simulink library "veh"  (Simulink 8.1)
settings: Solver=ode1  StartTime=0.0  StopTime=Inf  FixedStep=0.001  RelTol=1e-3
PostLoadFcn:
  | , if any(exist('dsrtsu_mdlpostloadfcn', 'file') == [2, 3, 6]), try dsrtsu_mdlpostloadfcn('Execute', bdroot); catch fprintf('Error in PostLoadFcn (dsrtsu_mdlpostloadfcn) for model "%s":\n %s\n', bdroot, lasterr); end, end,
undefined symbols (not defined in the file or in its folder): FALSE, KIFO_ACCRelSpeedNoTargets_kph, KIFO_LongAccelNoTargets_mps2, KIFO_RelSpeedNoTargets_kph, KIFO_TargetIdNoTargets_num, KIFO_XPositionNoTargets_m
libraries: hcu_lib x3, aco x1, mcs x1, vec x1, gim x1
settings Model: DSRTSU_INTERNAL_RTI_VER=450  DSRTSU_INTERNAL_RTI_TYPE=rti1401  RTICANMMDATA=struct('GeneralSetupData',struct('modelroot','D:\Projects\ELN150201\Repositories\Taiwan\trunk\AdasDragon\software\sw_development\arch\app\ifo','generalsettings',struct('filesettings',struct('destfolder',struct('Name','RTICANMM_FILES','Check',1),'buildfolder',struct('Name','.','Check',1),'AbsDestfolder',struct('Name','D:\Projects\ELN150201\Repositories\Taiwan\trunk\AdasDragon\software\sw_development\arch\app\ifo\RTICANMM_FILES'),'AbsBuildfolder',struct('Name','D:\Projects\ELN150201\Repositories\Taiwan\trunk\AdasDragon\software\sw_development\arch\app\ifo'))),'options',struct('addpaths',1,'rmpaths',1,'addtrcexclusion',logical(1),'cannavigator',struct('checkmonitoring',0),'show_usrtrc',0,'use_usrtrc',0),'advanced',struct('options',[1 1 1 1 1 1 1 1 1 1 1 1 1 1 1 1 1 1 1 1 1 1 1 1 1 1 1 1 1 1 1 1 1 1 1 1 1 1 1 1 1 1 1 1 1 1 1 1 1 1 1 1 1 1 1 1 1 1 1 1 1 1 1 1 1 1 1 1 1 1 1 1 1 1 1 1 1 1 1 1 1 1 1 1 1 1 1 1 1 1 1 1 1 1 1 1 1 1 1 1]),'MPSetup',{{}},'modelname','veh','block','veh'))  DSRTSU_INTERNAL_RTIFPGA=40  Creator=tescamilla  LastModifiedBy=AT015086

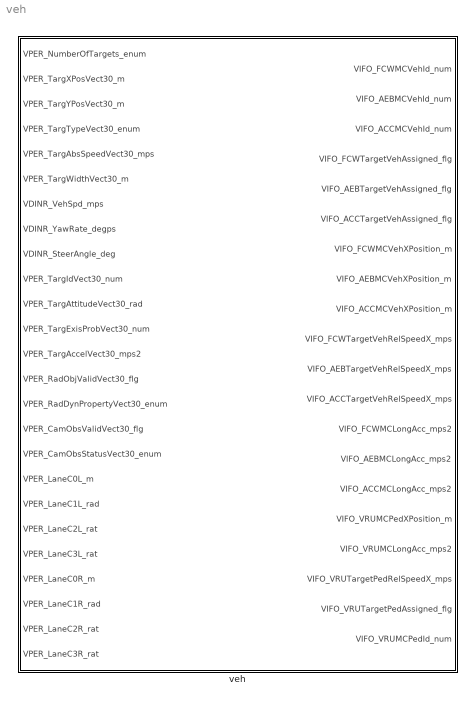
== system veh ==
  veh : Subsystem

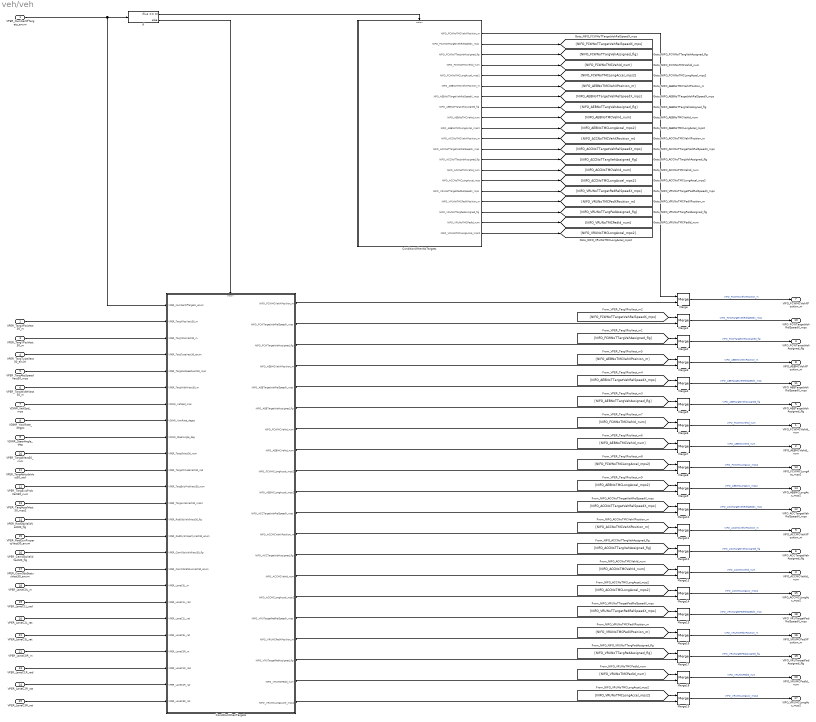
== system veh/veh ==
  VPER_NumberOfTargets_enum : Inport
  VPER_TargXPosVect30_m : Inport  Port=2
  VPER_TargYPosVect30_m : Inport  Port=3
  VPER_TargTypeVect30_enum : Inport  Port=4
  VPER_TargAbsSpeedVect30_mps : Inport  Port=5
  VPER_TargWidthVect30_m : Inport  Port=6
  VDINR_VehSpd_mps : Inport  Port=7
  VDINR_YawRate_degps : Inport  Port=8
  VDINR_SteerAngle_deg : Inport  Port=9
  VPER_TargIdVect30_num : Inport  Port=10
  VPER_TargAttitudeVect30_rad : Inport  Port=11
  VPER_TargExisProbVect30_num : Inport  Port=12
  VPER_TargAccelVect30_mps2 : Inport  Port=13
  VPER_RadObjValidVect30_flg : Inport  Port=14
  VPER_RadDynPropertyVect30_enum : Inport  Port=15
  VPER_CamObsValidVect30_flg : Inport  Port=16
  VPER_CamObsStatusVect30_enum : Inport  Port=17
  VPER_LaneC0L_m : Inport  Port=18
  VPER_LaneC1L_rad : Inport  Port=19
  VPER_LaneC2L_rat : Inport  Port=20
  VPER_LaneC3L_rat : Inport  Port=21
  VPER_LaneC0R_m : Inport  Port=22
  VPER_LaneC1R_rad : Inport  Port=23
  VPER_LaneC2R_rat : Inport  Port=24
  VPER_LaneC3R_rat : Inport  Port=25
  ConditionWhenNoTargets : Subsystem  TreatAsAtomicUnit=on
  ConditionWhenTargets : Subsystem  TreatAsAtomicUnit=on
  If : If  IfExpression=u1 == 0
  Merge : Merge  InitialOutput=KIFO_XPositionNoTargets_m
  Merge1 : Merge  InitialOutput=KIFO_RelSpeedNoTargets_kph
  Merge{6..19} (14 alike) : Merge  InitialOutput=KIFO_TargetIdNoTargets_num
  Merge2 : Merge  InitialOutput=FALSE
  Merge3 : Merge  InitialOutput=KIFO_XPositionNoTargets_m
  Merge4 : Merge  InitialOutput=KIFO_RelSpeedNoTargets_kph
  Merge5 : Merge  InitialOutput=FALSE
  VIFO_FCWMCVehId_num : Outport
  VIFO_AEBMCVehId_num : Outport  Port=2
  VIFO_ACCMCVehId_num : Outport  Port=3
  VIFO_FCWTargetVehAssigned_flg : Outport  Port=4
  VIFO_AEBTargetVehAssigned_flg : Outport  Port=5
  VIFO_ACCTargetVehAssigned_flg : Outport  Port=6
  VIFO_FCWMCVehXPosition_m : Outport  Port=7
  VIFO_AEBMCVehXPosition_m : Outport  Port=8
  VIFO_ACCMCVehXPosition_m : Outport  Port=9
  VIFO_FCWTargetVehRelSpeedX_mps : Outport  Port=10
  VIFO_AEBTargetVehRelSpeedX_mps : Outport  Port=11
  VIFO_ACCTargetVehRelSpeedX_mps : Outport  Port=12
  VIFO_FCWMCLongAcc_mps2 : Outport  Port=13
  VIFO_AEBMCLongAcc_mps2 : Outport  Port=14
  VIFO_ACCMCLongAcc_mps2 : Outport  Port=15
  VIFO_VRUMCPedXPosition_m : Outport  Port=16
  VIFO_VRUMCLongAcc_mps2 : Outport  Port=17
  VIFO_VRUTargetPedRelSpeedX_mps : Outport  Port=18
  VIFO_VRUTargetPedAssigned_flg : Outport  Port=19
  VIFO_VRUMCPedId_num : Outport  Port=20
  wires:
  ConditionWhenNoTargets/20(NIFO_VRUNoTMCLongAccel_mps2) -> [NIFO_VRUNoTMCLongAccel_mps2]
  ConditionWhenNoTargets/16(NIFO_VRUNoTTargetPedRelSpeedX_mps) -> [NIFO_VRUNoTTargetPedRelSpeedX_mps]
  ConditionWhenNoTargets/17(NIFO_VRUNoTMCPedXPosition_m) -> [NIFO_VRUNoTMCPedXPosition_m]
  ConditionWhenNoTargets/19(NIFO_VRUNoTMCPedId_num) -> [NIFO_VRUNoTMCPedId_num]
  ConditionWhenNoTargets/18(NIFO_VRUNoTTargPedAssigned_flg) -> [NIFO_VRUNoTTargPedAssigned_flg]
  [NIFO_VRUNoTMCLongAccel_mps2] -> Merge19/1
  Merge19/1 -> VIFO_VRUMCLongAcc_mps2/1  "VIFO_VRUMCLongAcc_mps2"
  ConditionWhenTargets/20(NIFO_VRUMCLongAccel_mps2) -> Merge19/2
  [NIFO_VRUNoTMCPedId_num] -> Merge18/1
  Merge18/1 -> VIFO_VRUMCPedId_num/1  "VIFO_VRUMCPedId_num"
  ConditionWhenTargets/19(NIFO_VRUMCPedId_num) -> Merge18/2
  [NIFO_VRUNoTTargPedAssigned_flg] -> Merge17/1
  Merge17/1 -> VIFO_VRUTargetPedAssigned_flg/1  "VIFO_VRUTargetPedAssigned_flg"
  ConditionWhenTargets/18(NIFO_VRUTargetPedAssigned_flg) -> Merge17/2
  [NIFO_VRUNoTMCPedXPosition_m] -> Merge16/1
  Merge16/1 -> VIFO_VRUMCPedXPosition_m/1  "VIFO_VRUMCPedXPosition_m"
  ConditionWhenTargets/17(NIFO_VRUMCPedXPosition_m) -> Merge16/2
  [NIFO_VRUNoTTargetPedRelSpeedX_mps] -> Merge15/1
  Merge15/1 -> VIFO_VRUTargetPedRelSpeedX_mps/1  "VIFO_VRUTargetPedRelSpeedX_mps"
  ConditionWhenTargets/16(NIFO_VRUTargetPedRelSpeedX_mps) -> Merge15/2
  [NIFO_ACCNoTMCLongAccel_mps2] -> Merge14/1
  Merge14/1 -> VIFO_ACCMCLongAcc_mps2/1  "VIFO_ACCMCLongAcc_mps2"
  ConditionWhenTargets/15(NIFO_ACCMCLongAccel_mps2) -> Merge14/2
  [NIFO_ACCNoTMCVehId_num] -> Merge13/1
  Merge13/1 -> VIFO_ACCMCVehId_num/1  "VIFO_ACCMCVehId_num"
  ConditionWhenTargets/14(NIFO_ACCMCVehId_num) -> Merge13/2
  [NIFO_ACCNoTTargVehAssigned_flg] -> Merge12/1
  Merge12/1 -> VIFO_ACCTargetVehAssigned_flg/1  "VIFO_ACCTargetVehAssigned_flg"
  ConditionWhenTargets/13(NIFO_ACCTargetVehAssigned_flg) -> Merge12/2
  [NIFO_ACCNoTMCVehXPosition_m] -> Merge11/1
  Merge11/1 -> VIFO_ACCMCVehXPosition_m/1  "VIFO_ACCMCVehXPosition_m"
  ConditionWhenTargets/12(NIFO_ACCMCVehXPosition_m) -> Merge11/2
  [NIFO_ACCNoTTargetVehRelSpeedX_mps] -> Merge10/1
  Merge10/1 -> VIFO_ACCTargetVehRelSpeedX_mps/1  "VIFO_ACCTargetVehRelSpeedX_mps"
  ConditionWhenTargets/11(NIFO_ACCTargetVehRelSpeedX_mps) -> Merge10/2
  ConditionWhenNoTargets/15(NIFO_ACCNoTMCLongAccel_mps) -> [NIFO_ACCNoTMCLongAccel_mps2]
  ConditionWhenNoTargets/14(NIFO_ACCNoTMCVehId_num) -> [NIFO_ACCNoTMCVehId_num]
  ConditionWhenNoTargets/13(NIFO_ACCNoTTargVehAssigned_flg) -> [NIFO_ACCNoTTargVehAssigned_flg]
  ConditionWhenNoTargets/12(NIFO_ACCNoTTargetVehRelSpeedX_mps) -> [NIFO_ACCNoTTargetVehRelSpeedX_mps]
  ConditionWhenNoTargets/11(NIFO_ACCNoTMCVehXPosition_m) -> [NIFO_ACCNoTMCVehXPosition_m]
  VPER_CamObsStatusVect30_enum/1 -> ConditionWhenTargets/17(VPER_CamObsStatusVect30_enum)
  VPER_CamObsValidVect30_flg/1 -> ConditionWhenTargets/16(VPER_CamObsValidVect30_flg)
  VPER_RadDynPropertyVect30_enum/1 -> ConditionWhenTargets/15(VPER_RadDynPropertyVect30_enum)
  VPER_RadObjValidVect30_flg/1 -> ConditionWhenTargets/14(VPER_RadObjValidVect30_flg)
  [NIFO_AEBNoTMCLongAccel_mps2] -> Merge9/1
  [NIFO_FCWNoTMCLongAccel_mps2] -> Merge8/1
  ConditionWhenNoTargets/10(NIFO_AEBNoTMCLongAccel_mps2) -> [NIFO_AEBNoTMCLongAccel_mps2]
  ConditionWhenNoTargets/5(NIFO_FCWNoTMCLongAccel_mps2) -> [NIFO_FCWNoTMCLongAccel_mps2]
  Merge9/1 -> VIFO_AEBMCLongAcc_mps2/1  "VIFO_AEBMCLongAcc_mps2"
  Merge8/1 -> VIFO_FCWMCLongAcc_mps2/1  "VIFO_FCWMCLongAcc_mps2"
  ConditionWhenTargets/10(NIFO_AEBMCLongAccel_mps2) -> Merge9/2
  ConditionWhenTargets/9(NIFO_FCWMCLongAccel_mps2) -> Merge8/2
  VPER_TargAccelVect30_mps2/1 -> ConditionWhenTargets/13(VPER_TargAccelVect30_mps2)
  VPER_TargXPosVect30_m/1 -> ConditionWhenTargets/2(VPER_TargXPosVect30_m)
  ConditionWhenNoTargets/9(NIFO_AEBNoTMCVehId_num) -> [NIFO_AEBNoTMCVehId_num]
  ConditionWhenNoTargets/4(NIFO_FCWNoTMCVehId_num) -> [NIFO_FCWNoTMCVehId_num]
  ConditionWhenTargets/7(NIFO_FCWMCVehId_num) -> Merge6/2
  [NIFO_FCWNoTMCVehId_num] -> Merge6/1
  ConditionWhenTargets/8(NIFO_AEBMCVehId_num) -> Merge7/2
  [NIFO_AEBNoTMCVehId_num] -> Merge7/1
  Merge6/1 -> VIFO_FCWMCVehId_num/1  "VIFO_FCWMCVehId_num"
  Merge7/1 -> VIFO_AEBMCVehId_num/1  "VIFO_AEBMCVehId_num"
  VPER_TargExisProbVect30_num/1 -> ConditionWhenTargets/12(VPER_TargExisProbVect30_num)
  VPER_TargAttitudeVect30_rad/1 -> ConditionWhenTargets/11(VPER_TargAttitudeVect30_rad)
  VPER_TargIdVect30_num/1 -> ConditionWhenTargets/10(VPER_TargIdVect30_num)
  [NIFO_AEBNoTMCVehXPosition_m] -> Merge3/1
  ConditionWhenNoTargets/6(NIFO_AEBNoTMCVehXPosition_m) -> [NIFO_AEBNoTMCVehXPosition_m]
  ConditionWhenNoTargets/7(NFO_AEBNoTTargetVehRelSpeedX_mps) -> [NIFO_AEBNoTTargetVehRelSpeedX_mps]
  ConditionWhenNoTargets/8(NIFO_AEBNoTTargVehAssigned_flg) -> [NIFO_AEBNoTTargVehAssigned_flg]
  ConditionWhenTargets/4(NIFO_AEBMCVehXPosition_m) -> Merge3/2
  ConditionWhenTargets/5(NIFO_AEBTargetVehRelSpeedX_mps) -> Merge4/2
  [NIFO_AEBNoTTargetVehRelSpeedX_mps] -> Merge4/1
  ConditionWhenTargets/6(NIFO_AEBTargetVehAssigned_flg) -> Merge5/2
  Merge3/1 -> VIFO_AEBMCVehXPosition_m/1  "VIFO_AEBMCVehXPosition_m"
  [NIFO_AEBNoTTargVehAssigned_flg] -> Merge5/1
  Merge4/1 -> VIFO_AEBTargetVehRelSpeedX_mps/1  "VIFO_AEBTargetVehRelSpeedX_mps"
  Merge5/1 -> VIFO_AEBTargetVehAssigned_flg/1  "VIFO_AEBTargetVehAssigned_flg"
  VDINR_SteerAngle_deg/1 -> ConditionWhenTargets/9(VDINR_SteerAngle_deg)
  VDINR_YawRate_degps/1 -> ConditionWhenTargets/8(VDINR_YawRate_degps)
  If/1 -> ConditionWhenNoTargets/Action
  If/2 -> ConditionWhenTargets/Action
  VPER_NumberOfTargets_enum/1 -> If/1, ConditionWhenTargets/1(VPER_NumberOfTargets_enum)
  VDINR_VehSpd_mps/1 -> ConditionWhenTargets/7(VDINR_VehSpd_mps)
  VPER_TargTypeVect30_enum/1 -> ConditionWhenTargets/4(VPER_TargTypeVect30_enum)
  VPER_TargYPosVect30_m/1 -> ConditionWhenTargets/3(VPER_TargYPosVect30_m)
  VPER_TargAbsSpeedVect30_mps/1 -> ConditionWhenTargets/5(VPER_TargAbsSpeedVect30_mps)
  VPER_TargWidthVect30_m/1 -> ConditionWhenTargets/6(VPER_TargWidthVect30_m)
  ConditionWhenNoTargets/1(NIFO_FCWNoTMCVehXPosition_m) -> Merge/1
  ConditionWhenNoTargets/2(NIFO_FCWNoTTargetVehRelSpeedX_mps) -> [NIFO_FCWNoTTargetVehRelSpeedX_mps]
  ConditionWhenTargets/1(NIFO_FCWMCVehXPosition_m) -> Merge/2
  ConditionWhenTargets/2(NIFO_FCWTargetVehRelSpeedX_mps) -> Merge1/2
  [NIFO_FCWNoTTargetVehRelSpeedX_mps] -> Merge1/1
  ConditionWhenTargets/3(NIFO_FCWTargetVehAssigned_flg) -> Merge2/2
  ConditionWhenNoTargets/3(NIFO_FCWNoTTargVehAssigned_flg) -> [NIFO_FCWNoTTargVehAssigned_flg]
  Merge/1 -> VIFO_FCWMCVehXPosition_m/1  "VIFO_FCWMCVehXPosition_m"
  [NIFO_FCWNoTTargVehAssigned_flg] -> Merge2/1
  Merge1/1 -> VIFO_FCWTargetVehRelSpeedX_mps/1  "VIFO_FCWTargetVehRelSpeedX_mps"
  Merge2/1 -> VIFO_FCWTargetVehAssigned_flg/1  "VIFO_FCWTargetVehAssigned_flg"
  VPER_LaneC0L_m/1 -> ConditionWhenTargets/18(VPER_LaneC0L_m)
  VPER_LaneC1L_rad/1 -> ConditionWhenTargets/19(VPER_LaneC1L_rad)
  VPER_LaneC2L_rat/1 -> ConditionWhenTargets/20(VPER_LaneC2L_rat)
  VPER_LaneC3L_rat/1 -> ConditionWhenTargets/21(VPER_LaneC3L_rat)
  VPER_LaneC0R_m/1 -> ConditionWhenTargets/22(VPER_LaneC0R_m)
  VPER_LaneC1R_rad/1 -> ConditionWhenTargets/23(VPER_LaneC1R_rad)
  VPER_LaneC2R_rat/1 -> ConditionWhenTargets/24(VPER_LaneC2R_rat)
  VPER_LaneC3R_rat/1 -> ConditionWhenTargets/25(VPER_LaneC3R_rat)

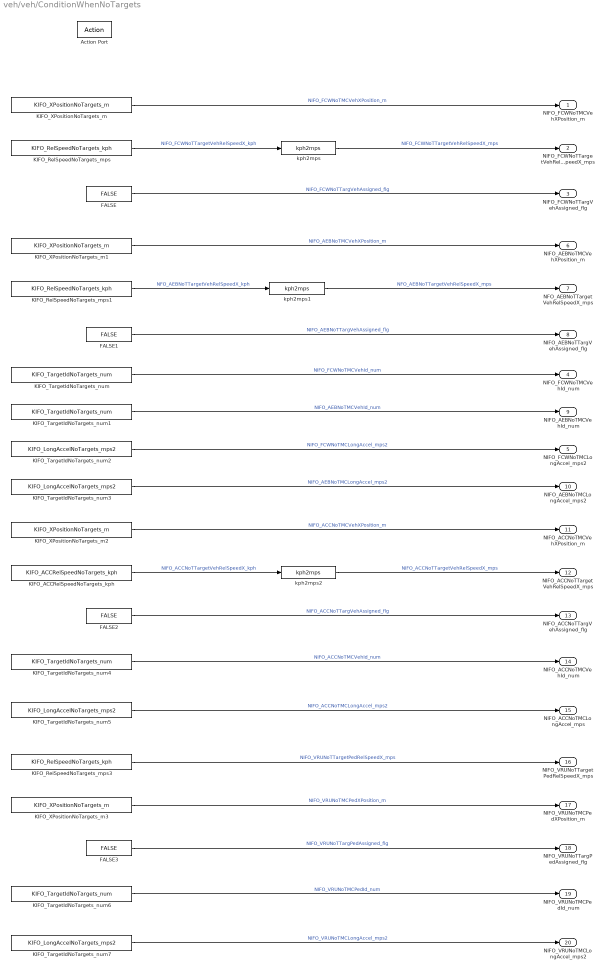
== system veh/veh/ConditionWhenNoTargets ==
  Action Port : ActionPort
  FALSE{,1..3} (4 alike) : Constant  Value=FALSE
  KIFO_ACCRelSpeedNoTargets_kph : Constant  Value=KIFO_ACCRelSpeedNoTargets_kph
  KIFO_RelSpeedNoTargets_mps : Constant  Value=KIFO_RelSpeedNoTargets_kph
  KIFO_RelSpeedNoTargets_mps1 : Constant  Value=KIFO_RelSpeedNoTargets_kph
  KIFO_RelSpeedNoTargets_mps3 : Constant  Value=KIFO_RelSpeedNoTargets_kph
  KIFO_TargetIdNoTargets_num{,1,4,6} (4 alike) : Constant  Value=KIFO_TargetIdNoTargets_num
  KIFO_TargetIdNoTargets_num{2..3,5,7} (4 alike) : Constant  Value=KIFO_LongAccelNoTargets_mps2
  KIFO_XPositionNoTargets_m{,1..3} (4 alike) : Constant  Value=KIFO_XPositionNoTargets_m
  kph2mps : hcu_lib/kph2mps
  kph2mps1 : hcu_lib/kph2mps
  kph2mps2 : hcu_lib/kph2mps
  NIFO_FCWNoTMCVehXPosition_m : Outport
  NIFO_FCWNoTTargetVehRelSpeedX_mps : Outport  Port=2
  NIFO_FCWNoTTargVehAssigned_flg : Outport  Port=3
  NIFO_FCWNoTMCVehId_num : Outport  Port=4
  NIFO_FCWNoTMCLongAccel_mps2 : Outport  Port=5
  NIFO_AEBNoTMCVehXPosition_m : Outport  Port=6
  NFO_AEBNoTTargetVehRelSpeedX_mps : Outport  Port=7
  NIFO_AEBNoTTargVehAssigned_flg : Outport  Port=8
  NIFO_AEBNoTMCVehId_num : Outport  Port=9
  NIFO_AEBNoTMCLongAccel_mps2 : Outport  Port=10
  NIFO_ACCNoTMCVehXPosition_m : Outport  Port=11
  NIFO_ACCNoTTargetVehRelSpeedX_mps : Outport  Port=12
  NIFO_ACCNoTTargVehAssigned_flg : Outport  Port=13
  NIFO_ACCNoTMCVehId_num : Outport  Port=14
  NIFO_ACCNoTMCLongAccel_mps : Outport  Port=15
  NIFO_VRUNoTTargetPedRelSpeedX_mps : Outport  Port=16
  NIFO_VRUNoTMCPedXPosition_m : Outport  Port=17
  NIFO_VRUNoTTargPedAssigned_flg : Outport  Port=18
  NIFO_VRUNoTMCPedId_num : Outport  Port=19
  NIFO_VRUNoTMCLongAccel_mps2 : Outport  Port=20
  wires:
  KIFO_TargetIdNoTargets_num7/1 -> NIFO_VRUNoTMCLongAccel_mps2/1  "NIFO_VRUNoTMCLongAccel_mps2"
  KIFO_TargetIdNoTargets_num6/1 -> NIFO_VRUNoTMCPedId_num/1  "NIFO_VRUNoTMCPedId_num"
  FALSE3/1 -> NIFO_VRUNoTTargPedAssigned_flg/1  "NIFO_VRUNoTTargPedAssigned_flg"
  KIFO_XPositionNoTargets_m3/1 -> NIFO_VRUNoTMCPedXPosition_m/1  "NIFO_VRUNoTMCPedXPosition_m"
  KIFO_RelSpeedNoTargets_mps3/1 -> NIFO_VRUNoTTargetPedRelSpeedX_mps/1  "NIFO_VRUNoTTargetPedRelSpeedX_mps"
  KIFO_TargetIdNoTargets_num5/1 -> NIFO_ACCNoTMCLongAccel_mps/1  "NIFO_ACCNoTMCLongAccel_mps2"
  KIFO_TargetIdNoTargets_num4/1 -> NIFO_ACCNoTMCVehId_num/1  "NIFO_ACCNoTMCVehId_num"
  FALSE2/1 -> NIFO_ACCNoTTargVehAssigned_flg/1  "NIFO_ACCNoTTargVehAssigned_flg"
  kph2mps2/1 -> NIFO_ACCNoTTargetVehRelSpeedX_mps/1  "NIFO_ACCNoTTargetVehRelSpeedX_mps"
  KIFO_ACCRelSpeedNoTargets_kph/1 -> kph2mps2/1  "NIFO_ACCNoTTargetVehRelSpeedX_kph"
  KIFO_XPositionNoTargets_m2/1 -> NIFO_ACCNoTMCVehXPosition_m/1  "NIFO_ACCNoTMCVehXPosition_m"
  KIFO_TargetIdNoTargets_num3/1 -> NIFO_AEBNoTMCLongAccel_mps2/1  "NIFO_AEBNoTMCLongAccel_mps2"
  KIFO_TargetIdNoTargets_num2/1 -> NIFO_FCWNoTMCLongAccel_mps2/1  "NIFO_FCWNoTMCLongAccel_mps2"
  kph2mps1/1 -> NFO_AEBNoTTargetVehRelSpeedX_mps/1  "NFO_AEBNoTTargetVehRelSpeedX_mps"
  kph2mps/1 -> NIFO_FCWNoTTargetVehRelSpeedX_mps/1  "NIFO_FCWNoTTargetVehRelSpeedX_mps"
  KIFO_TargetIdNoTargets_num1/1 -> NIFO_AEBNoTMCVehId_num/1  "NIFO_AEBNoTMCVehId_num"
  KIFO_TargetIdNoTargets_num/1 -> NIFO_FCWNoTMCVehId_num/1  "NIFO_FCWNoTMCVehId_num"
  KIFO_XPositionNoTargets_m1/1 -> NIFO_AEBNoTMCVehXPosition_m/1  "NIFO_AEBNoTMCVehXPosition_m"
  KIFO_RelSpeedNoTargets_mps1/1 -> kph2mps1/1  "NFO_AEBNoTTargetVehRelSpeedX_kph"
  FALSE1/1 -> NIFO_AEBNoTTargVehAssigned_flg/1  "NIFO_AEBNoTTargVehAssigned_flg"
  KIFO_XPositionNoTargets_m/1 -> NIFO_FCWNoTMCVehXPosition_m/1  "NIFO_FCWNoTMCVehXPosition_m"
  KIFO_RelSpeedNoTargets_mps/1 -> kph2mps/1  "NIFO_FCWNoTTargetVehRelSpeedX_kph"
  FALSE/1 -> NIFO_FCWNoTTargVehAssigned_flg/1  "NIFO_FCWNoTTargVehAssigned_flg"

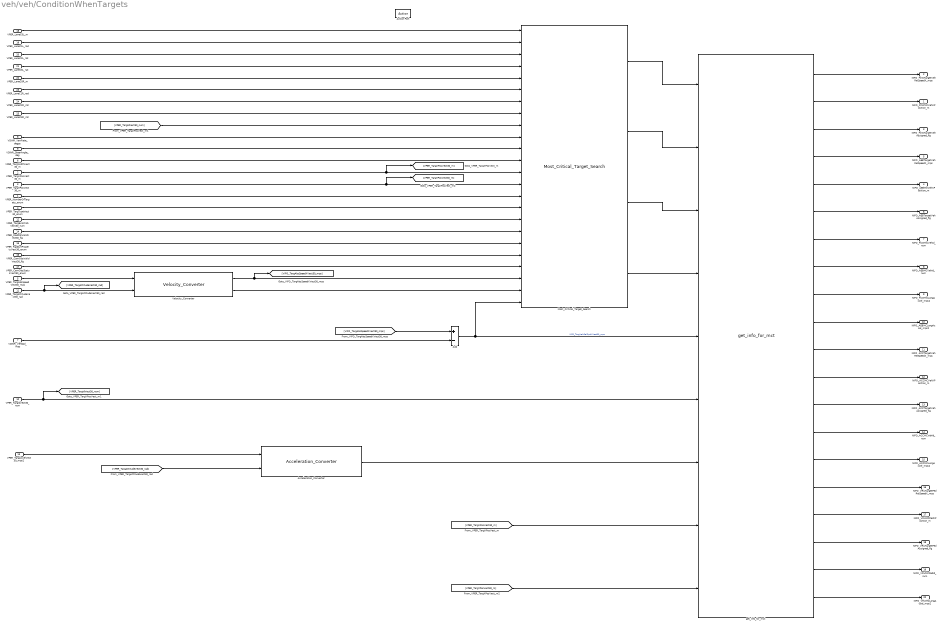
== system veh/veh/ConditionWhenTargets ==
  VPER_NumberOfTargets_enum : Inport
  VPER_TargXPosVect30_m : Inport  Port=2
  VPER_TargYPosVect30_m : Inport  Port=3
  VPER_TargTypeVect30_enum : Inport  Port=4
  VPER_TargAbsSpeedVect30_mps : Inport  Port=5
  VPER_TargWidthVect30_m : Inport  Port=6
  VDINR_VehSpd_mps : Inport  Port=7
  VDINR_YawRate_degps : Inport  Port=8
  VDINR_SteerAngle_deg : Inport  Port=9
  VPER_TargIdVect30_num : Inport  Port=10
  VPER_TargAttitudeVect30_rad : Inport  Port=11
  VPER_TargExisProbVect30_num : Inport  Port=12
  VPER_TargAccelVect30_mps2 : Inport  Port=13
  VPER_RadObjValidVect30_flg : Inport  Port=14
  VPER_RadDynPropertyVect30_enum : Inport  Port=15
  VPER_CamObsValidVect30_flg : Inport  Port=16
  VPER_CamObsStatusVect30_enum : Inport  Port=17
  VPER_LaneC0L_m : Inport  Port=18
  VPER_LaneC1L_rad : Inport  Port=19
  VPER_LaneC2L_rat : Inport  Port=20
  VPER_LaneC3L_rat : Inport  Port=21
  VPER_LaneC0R_m : Inport  Port=22
  VPER_LaneC1R_rad : Inport  Port=23
  VPER_LaneC2R_rat : Inport  Port=24
  VPER_LaneC3R_rat : Inport  Port=25
  Action Port : ActionPort
  Acceleration_Converter : aco/Acceleration_Converter
  Add : Sum  Inputs=+-
  Most_Critical_Target_Search : mcs/Most_Critical_Target_Search
  Velocity_Converter : vec/Velocity_Converter
  get_info_for_mct : gim/get_info_for_mct
  NIFO_FCWMCVehXPosition_m : Outport
  NIFO_FCWTargetVehRelSpeedX_mps : Outport  Port=2
  NIFO_FCWTargetVehAssigned_flg : Outport  Port=3
  NIFO_AEBMCVehXPosition_m : Outport  Port=4
  NIFO_AEBTargetVehRelSpeedX_mps : Outport  Port=5
  NIFO_AEBTargetVehAssigned_flg : Outport  Port=6
  NIFO_FCWMCVehId_num : Outport  Port=7
  NIFO_AEBMCVehId_num : Outport  Port=8
  NIFO_FCWMCLongAccel_mps2 : Outport  Port=9
  NIFO_AEBMCLongAccel_mps2 : Outport  Port=10
  NIFO_ACCTargetVehRelSpeedX_mps : Outport  Port=11
  NIFO_ACCMCVehXPosition_m : Outport  Port=12
  NIFO_ACCTargetVehAssigned_flg : Outport  Port=13
  NIFO_ACCMCVehId_num : Outport  Port=14
  NIFO_ACCMCLongAccel_mps2 : Outport  Port=15
  NIFO_VRUTargetPedRelSpeedX_mps : Outport  Port=16
  NIFO_VRUMCPedXPosition_m : Outport  Port=17
  NIFO_VRUTargetPedAssigned_flg : Outport  Port=18
  NIFO_VRUMCPedId_num : Outport  Port=19
  NIFO_VRUMCLongAccel_mps2 : Outport  Port=20
  wires:
  get_info_for_mct/20 -> NIFO_VRUMCLongAccel_mps2/1
  get_info_for_mct/19 -> NIFO_VRUMCPedId_num/1
  get_info_for_mct/18 -> NIFO_VRUTargetPedAssigned_flg/1
  get_info_for_mct/17 -> NIFO_VRUMCPedXPosition_m/1
  get_info_for_mct/16 -> NIFO_VRUTargetPedRelSpeedX_mps/1
  Most_Critical_Target_Search/4 -> get_info_for_mct/4
  [VIFO_TargAbsSpeedXVect30_mps] -> Add/1
  get_info_for_mct/15 -> NIFO_ACCMCLongAccel_mps2/1
  get_info_for_mct/14 -> NIFO_ACCMCVehId_num/1
  get_info_for_mct/13 -> NIFO_ACCTargetVehAssigned_flg/1
  Most_Critical_Target_Search/3 -> get_info_for_mct/3
  get_info_for_mct/12 -> NIFO_ACCMCVehXPosition_m/1
  get_info_for_mct/11 -> NIFO_ACCTargetVehRelSpeedX_mps/1
  VPER_CamObsStatusVect30_enum/1 -> Most_Critical_Target_Search/21
  Acceleration_Converter/1 -> get_info_for_mct/7
  [VPER_TargAttitudeVect30_rad] -> Acceleration_Converter/2
  VPER_CamObsValidVect30_flg/1 -> Most_Critical_Target_Search/20
  VPER_RadDynPropertyVect30_enum/1 -> Most_Critical_Target_Search/19
  VPER_RadObjValidVect30_flg/1 -> Most_Critical_Target_Search/18
  get_info_for_mct/10 -> NIFO_AEBMCLongAccel_mps2/1
  get_info_for_mct/9 -> NIFO_FCWMCLongAccel_mps2/1
  VPER_TargAccelVect30_mps2/1 -> Acceleration_Converter/1
  [VPER_TargIdVect30_num] -> Most_Critical_Target_Search/9
  Velocity_Converter/2 -> Most_Critical_Target_Search/23
  VPER_TargAttitudeVect30_rad/1 -> [VPER_TargAttitudeVect30_rad], Velocity_Converter/2
  Velocity_Converter/1 -> Most_Critical_Target_Search/22, [VIFO_TargAbsSpeedXVect30_mps]
  get_info_for_mct/8 -> NIFO_AEBMCVehId_num/1
  get_info_for_mct/7 -> NIFO_FCWMCVehId_num/1
  VPER_TargIdVect30_num/1 -> get_info_for_mct/6, [VPER_TargIdVect30_num]
  VPER_TargExisProbVect30_num/1 -> Most_Critical_Target_Search/17
  Most_Critical_Target_Search/2 -> get_info_for_mct/2
  Most_Critical_Target_Search/1 -> get_info_for_mct/1
  VPER_TargTypeVect30_enum/1 -> Most_Critical_Target_Search/16
  VPER_NumberOfTargets_enum/1 -> Most_Critical_Target_Search/15
  VPER_TargYPosVect30_m/1 -> [VPER_TargYPosVect30_m], Most_Critical_Target_Search/14
  VPER_TargXPosVect30_m/1 -> Most_Critical_Target_Search/13, [VPER_TargXPosVect30_m]
  VPER_TargWidthVect30_m/1 -> Most_Critical_Target_Search/12
  VDINR_SteerAngle_deg/1 -> Most_Critical_Target_Search/11
  VDINR_YawRate_degps/1 -> Most_Critical_Target_Search/10
  get_info_for_mct/6 -> NIFO_AEBTargetVehAssigned_flg/1
  get_info_for_mct/5 -> NIFO_AEBMCVehXPosition_m/1
  get_info_for_mct/4 -> NIFO_AEBTargetVehRelSpeedX_mps/1
  [VPER_TargXPosVect30_m] -> get_info_for_mct/8
  get_info_for_mct/3 -> NIFO_FCWTargetVehAssigned_flg/1
  get_info_for_mct/2 -> NIFO_FCWMCVehXPosition_m/1
  get_info_for_mct/1 -> NIFO_FCWTargetVehRelSpeedX_mps/1
  Add/1 -> Most_Critical_Target_Search/24, get_info_for_mct/5  "VIFO_TargVehRelSpdXVect30_mps"
  VPER_TargAbsSpeedVect30_mps/1 -> Velocity_Converter/1
  VDINR_VehSpd_mps/1 -> Add/2
  VPER_LaneC2R_rat/1 -> Most_Critical_Target_Search/7
  VPER_LaneC3R_rat/1 -> Most_Critical_Target_Search/8
  VPER_LaneC1R_rad/1 -> Most_Critical_Target_Search/6
  VPER_LaneC0R_m/1 -> Most_Critical_Target_Search/5
  VPER_LaneC3L_rat/1 -> Most_Critical_Target_Search/4
  VPER_LaneC2L_rat/1 -> Most_Critical_Target_Search/3
  VPER_LaneC1L_rad/1 -> Most_Critical_Target_Search/2
  VPER_LaneC0L_m/1 -> Most_Critical_Target_Search/1
  [VPER_TargYPosVect30_m] -> get_info_for_mct/9
